simulink model "p2_rcrc_frf_sldrt"  (R2024a)
settings: Solver=ode3  StartTime=0.0  StopTime=10  FixedStep=Ts  RelTol=1e-3
PostLoadFcn:
  | try
  | if isempty(which('ZHAWcbfcn'));
  | callback_fid07124=fopen('ZHAWcbfcn.m','w');
  | [~]=fprintf(callback_fid07124,'%s',get_param([bdroot,'/ Setup SLDRT'],'ClipboardFcn'));
  | [~]=fclose(callback_fid07124);
  | setpref('ZHAW_SLDRT_lib','cb_fcn',which('ZHAWcbfcn'))
  | clear callback_fid07124
  | end
  | catch
  | clear callback_fid07124
  | end
  | Ts=eval(get_param([bdroot,'/ Setup SLDRT'],'Ts'));
InitFcn:
  | Ts=eval(get_param([bdroot,'/ Setup SLDRT'],'Ts'));
undefined symbols (not defined in the file or in its folder): National_Instruments, PCIe
libraries: sldrtlib x3
(part 2 of 2)

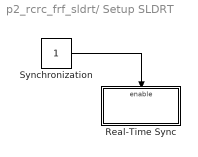
== system p2_rcrc_frf_sldrt/ Setup SLDRT ==
  Real-Time Sync : Subsystem
  Synchronization : Constant
  wires:
  Synchronization/1 -> Real-Time Sync/Enable

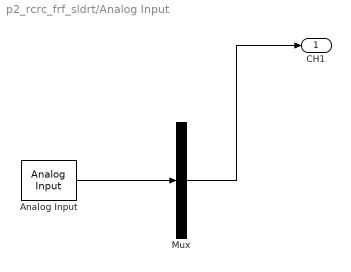
== system p2_rcrc_frf_sldrt/Analog Input ==
  Analog Input : sldrtlib/Analog Input  SampleTime=Ts  MaxMissedTicks=10  ShowMissedTicks=off  YieldWhenWaiting=off  DrvName=National_Instruments/PCIe-6321  DrvAddress=4294967295  DrvOptions="[1  0  0  2  2  2  2]"  Channels=ch_list  RangeMode=1  VoltRange=1  DataType=1
      settings: AttributesFormatString=National Instruments\nPCIe-6321 [auto]
  Mux : Demux  Outputs=1
  CH1 : Outport  VectorParamsAs1DForOutWhenUnconnected=off
  wires:
  Mux/1 -> CH1/1
  Analog Input/1 -> Mux/1

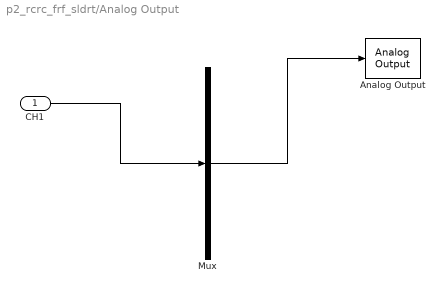
== system p2_rcrc_frf_sldrt/Analog Output ==
  CH1 : Inport
  Analog Output : sldrtlib/Analog Output  SampleTime=Ts  MaxMissedTicks=10  ShowMissedTicks=off  YieldWhenWaiting=off  DrvName=National_Instruments/PCIe-6321  DrvAddress=4294967295  DrvOptions="[1  0  0  2  2  2  2]"  Channels=ch_list  RangeMode=1  VoltRange=1  InitialValue=0  FinalValue=0
      settings: AttributesFormatString=National Instruments\nPCIe-6321 [auto]
  Mux : Mux  Inputs=1
  wires:
  Mux/1 -> Analog Output/1
  CH1/1 -> Mux/1

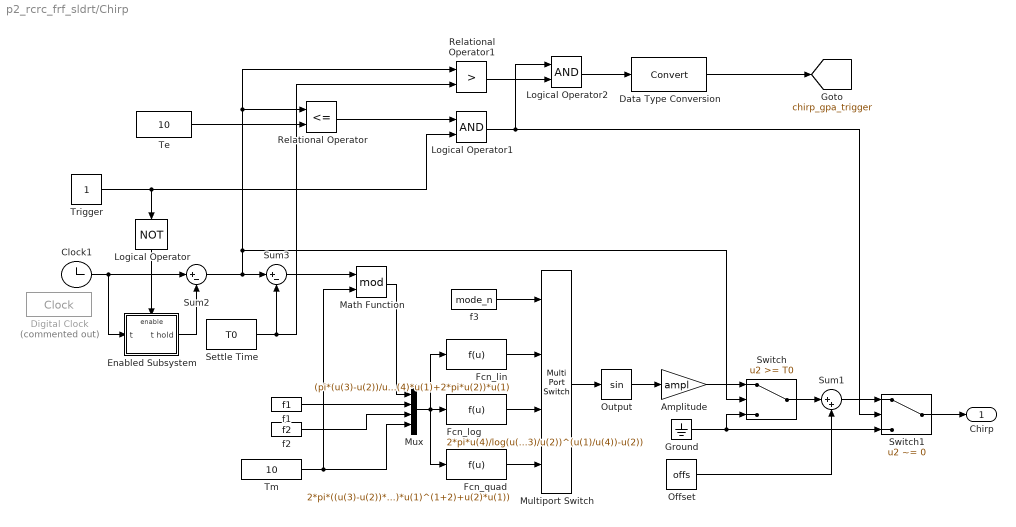
== system p2_rcrc_frf_sldrt/Chirp ==
  Amplitude : Gain  Gain=ampl
  Clock1 : Clock
      settings: DisableCoverage=on
  Data Type Conversion : DataTypeConversion  SaturateOnIntegerOverflow=off  RndMeth=Floor
  Digital Clock : DigitalClock  Commented=on  SampleTime=Ts
  Enabled Subsystem : Subsystem  TreatAsAtomicUnit=on
  Fcn_lin : Fcn  Expr=(pi*(u(3)-u(2))/u(4)*u(1)+2*pi*u(2))*u(1)
  Fcn_log : Fcn  Expr=2*pi*u(4)/log(u(3)/u(2))*(u(2)*(u(3)/u(2))^(u(1)/u(4))-u(2))
  Fcn_quad : Fcn  Expr=2*pi*((u(3)-u(2))*u(4)^(-2)/(1+2)*u(1)^(1+2)+u(2)*u(1))
  Ground : Ground
  Logical Operator : Logic  Operator=NOT  AllPortsSameDT=off  OutDataTypeStr=boolean
  Logical Operator1 : Logic  AllPortsSameDT=off
  Logical Operator2 : Logic  AllPortsSameDT=off
  Math Function : Math  Operator=mod  SignedPower=on
  Multiport Switch : MultiPortSwitch  SaturateOnIntegerOverflow=off  InputSameDT=off
  Mux : Mux
  Offset : Constant  Value=offs
  Output : Trigonometry
  Relational Operator : RelationalOperator  Operator=<=  RndMeth=Simplest  InputSameDT=off
  Relational Operator1 : RelationalOperator  Operator=>  RndMeth=Simplest  InputSameDT=off
  Settle Time : Constant  Value=T0
  Sum1 : Sum  Inputs=|++
  Sum2 : Sum  Inputs=|+-
  Sum3 : Sum  Inputs=|+-
  Switch : Switch  Threshold=T0  SaturateOnIntegerOverflow=off  InputSameDT=off
  Switch1 : Switch  Criteria=u2 ~= 0  SaturateOnIntegerOverflow=off  InputSameDT=off
  Te : Constant  Value=10
  Tm : Constant  Value=10
  Trigger : Constant
  f1 : Constant  Value=f1
  f2 : Constant  Value=f2
  f3 : Constant  Value=mode_n
  Chirp : Outport  VectorParamsAs1DForOutWhenUnconnected=off
  tag scope: chirp_gpa_trigger=global
  wires:
  Te/1 -> Relational Operator/2
  Logical Operator/1 -> Enabled Subsystem/Enable
  Enabled Subsystem/1(t hold) -> Sum2/2
  Trigger/1 -> Logical Operator1/2, Logical Operator/1
  f3/1 -> Multiport Switch/1
  Fcn_lin/1 -> Multiport Switch/2
  Fcn_log/1 -> Multiport Switch/3
  Fcn_quad/1 -> Multiport Switch/4
  Multiport Switch/1 -> Output/1
  Math Function/1 -> Mux/1
  f2/1 -> Mux/3
  f1/1 -> Mux/2
  Mux/1 -> Fcn_log/1, Fcn_lin/1, Fcn_quad/1
  Clock1/1 -> Enabled Subsystem/1(t), Sum2/1
  Output/1 -> Amplitude/1
  Offset/1 -> Sum1/2
  Sum3/1 -> Math Function/1
  Tm/1 -> Mux/4, Math Function/2
  Switch/1 -> Sum1/1
  Amplitude/1 -> Switch/1
  Ground/1 -> Switch1/3, Switch/3
  Settle Time/1 -> Relational Operator1/2, Sum3/2
  Sum2/1 -> Switch/2, Relational Operator1/1, Relational Operator/1, Sum3/1
  Switch1/1 -> Chirp/1
  Sum1/1 -> Switch1/1
  Relational Operator/1 -> Logical Operator1/1
  Logical Operator1/1 -> Logical Operator2/1, Switch1/2
  Logical Operator2/1 -> Data Type Conversion/1
  Data Type Conversion/1 -> [chirp_gpa_trigger]
  Relational Operator1/1 -> Logical Operator2/2

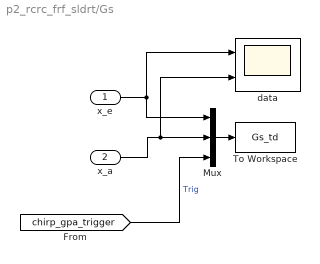
== system p2_rcrc_frf_sldrt/Gs ==
  x_e : Inport
  x_a : Inport  Port=2
  Mux : Mux  Inputs=3
  To Workspace : ToWorkspace  VariableName=Gs_td  SaveFormat=Structure With Time  SampleTime=Ts
  data : Scope  NumInputPorts=2
      settings: CopyFcn=try ZHAWcbfcn('copyScope'); end  NameChangeFcn=try ZHAWcbfcn('namechangeScope'); end
  wires:
  x_e/1 -> data/1, Mux/1
  x_a/1 -> data/2, Mux/2
  Mux/1 -> To Workspace/1
  [chirp_gpa_trigger] -> Mux/3  "Trig"

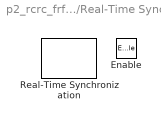
== system p2_rcrc_frf_sldrt/ Setup SLDRT/Real-Time Sync ==
  Enable : EnablePort
  Real-Time Synchronization : sldrtlib/Real-Time Synchronization  SampleTime=Ts  MaxMissedTicks=inf  ShowMissedTicks=off  YieldWhenWaiting=off

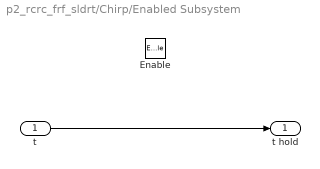
== system p2_rcrc_frf_sldrt/Chirp/Enabled Subsystem ==
  t : Inport
  Enable : EnablePort
  t hold : Outport  VectorParamsAs1DForOutWhenUnconnected=off
  wires:
  t/1 -> t hold/1
